simulink model "b747cl"  (Simulink 3.00)
settings: Solver=FixedStepDiscrete  StartTime=0.0  StopTime=Inf  RelTol=1e-3
libraries: simulink3 x2, airlib x1
settings Model: SaveTime=off  SaveOutput=off  ExtModeTrigMode=normal  ExtModeArmWhenConnect=on  LastModifiedBy=gcampa

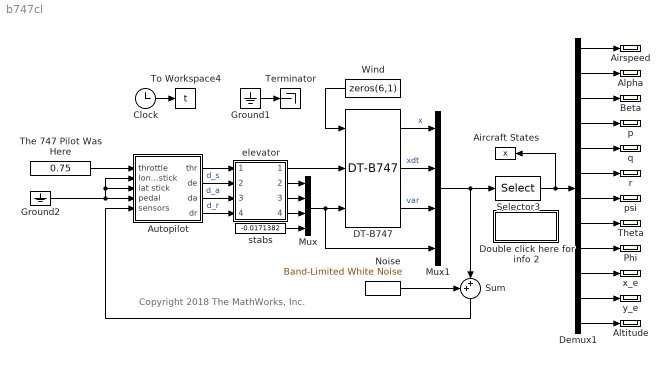
== system b747cl ==
  note: Copyright 2018 The MathWorks, Inc.
  Aircraft States : ToWorkspace  VariableName=x  SampleTime=0.05  SaveFormat=Matrix
      settings: Buffer=1000
  Airspeed : Scope
      settings: TimeRange=100  YMin=142.641  YMax=157.655  SaveToWorkspace=off  SaveName=ScopeData5
  Alpha : Scope
      settings: TimeRange=100  YMin=0.044176  YMax=0.0488262  SaveToWorkspace=off  SaveName=ScopeData4
  Altitude : Scope
      settings: TimeRange=100  YMin=57.9499  YMax=64.0499  SaveToWorkspace=off  SaveName=ScopeData15
  Autopilot : Subsystem
  Beta : Scope
      settings: TimeRange=100  YMin=0  YMax=250000  SaveToWorkspace=off  SaveName=ScopeData6
  Clock : Clock
      settings: DisplayTime=off  Decimation=10
  DT-B747 : airlib/DT-B747  GM1="[8.32   59.74   510.95   24675560  44876980   67383260   0   1315126  0   288772  0.05]"  CD_wind="[0.0164  0.2  0  0  0]"  CL_wind="[0.21  4.4  6.6  0.32  0.7]"  Cm_body="[0  -1   -20.5    -1.3    -2.7]"  CY_body="[0   -0.9    0     0     -0    0.12]"  Cl_body="[0    -0.16    -0.34   0.13    -0.013    0.008]"  Cn_body="[0    0.16   -0.026    -0.28     -0.0018   -0.1]"  x0="[150.148  0.0464959 0   0 0 0   0 0.0464959 0   0 0 61]"
  Demux1 : Demux  Outputs=12
  Double click here for info 2 : Subsystem
      mask Display: disp('Output\nSignals')
  Ground1 : Ground
  Ground2 : Ground
  Mux : Mux  Inputs=4
      settings: DisplayOption=none
  Mux1 : Mux  Inputs=[12 12 12 4]
      settings: DisplayOption=none
  Noise : simulink3/Sources/Band-Limited White Noise  Cov=[1e-7*ones(1,6) 1e-10*ones(1,3) zeros(1,31)]  Ts=0.05  seed=1:40
  Phi : Scope
      settings: TimeRange=100  YMin=-0.0002446  YMax=-0.0002438  SaveToWorkspace=off  SaveName=ScopeData12
  Selector3 : Selector  Elements=1:12  InputPortWidth=40
  Sum : Sum  Orientation=down  Inputs=++|  SaturateOnIntegerOverflow=on
  Terminator : Terminator
  The 747 Pilot Was Here : Constant  Value=0.75
  Theta : Scope
      settings: TimeRange=300  YMin=0.0463  YMax=0.0467  SaveToWorkspace=off  SaveName=ScopeData11
  To Workspace4 : ToWorkspace  VariableName=t  SampleTime=0.05  SaveFormat=Matrix
      settings: Buffer=1000
  Wind : Constant  Orientation=left  Value=zeros(6,1)
  elevator : Subsystem
      mask Display: disp('Cable &\nactuator\ndynamics')
  p : Scope
      settings: TimeRange=100  YMin=0  YMax=250000  SaveToWorkspace=off  SaveName=ScopeData7
  psi : Scope
      settings: TimeRange=100  YMin=0  YMax=250000  SaveToWorkspace=off  SaveName=ScopeData10
  q : Scope
      settings: TimeRange=100  YMin=0  YMax=250000  SaveToWorkspace=off  SaveName=ScopeData8
  r : Scope
      settings: TimeRange=100  YMin=0  YMax=250000  SaveToWorkspace=off  SaveName=ScopeData9
  stabs : Constant  Value=-0.0171382
  x_e : Scope
      settings: TimeRange=100  YMin=0  YMax=250000  SaveToWorkspace=off  SaveName=ScopeData13
  y_e : Scope
      settings: TimeRange=100  YMin=0  YMax=250000  SaveToWorkspace=off  SaveName=ScopeData14
  wires:
  elevator/3(deltaa) -> Mux/2
  elevator/4(deltar) -> Mux/3
  elevator/2(deltae) -> Mux/1
  Autopilot/2(de) -> elevator/2(D_elv)  "d_s"
  Autopilot/3(da) -> elevator/3(D_ail)  "d_a"
  Autopilot/4(dr) -> elevator/4(D_rud)  "d_r"
  Mux/1 -> Mux1/4, DT-B747/3
  elevator/1(throttle) -> DT-B747/2
  Mux1/1 -> Selector3/1, Sum/2
  Selector3/1 -> Demux1/1, Aircraft States/1
  Demux1/1 -> Airspeed/1
  Demux1/2 -> Alpha/1
  Demux1/3 -> Beta/1
  Demux1/4 -> p/1
  Demux1/5 -> q/1
  Demux1/6 -> r/1
  Demux1/7 -> psi/1
  Demux1/8 -> Theta/1
  Demux1/9 -> Phi/1
  Demux1/10 -> x_e/1
  Demux1/11 -> y_e/1
  Demux1/12 -> Altitude/1
  Autopilot/1(thr) -> elevator/1(D_thr)
  Clock/1 -> To Workspace4/1
  stabs/1 -> Mux/4
  Wind/1 -> DT-B747/1
  DT-B747/1 -> Mux1/1  "x"
  DT-B747/2 -> Mux1/2  "xdt"
  DT-B747/3 -> Mux1/3  "var"
  The 747 Pilot Was Here/1 -> Autopilot/1(throttle)
  Ground2/1 -> Autopilot/4(pedal), Autopilot/3(lat stick), Autopilot/2(long stick)
  Sum/1 -> Autopilot/5(sensors)
  Noise/1 -> Sum/1
  Ground1/1 -> Terminator/1

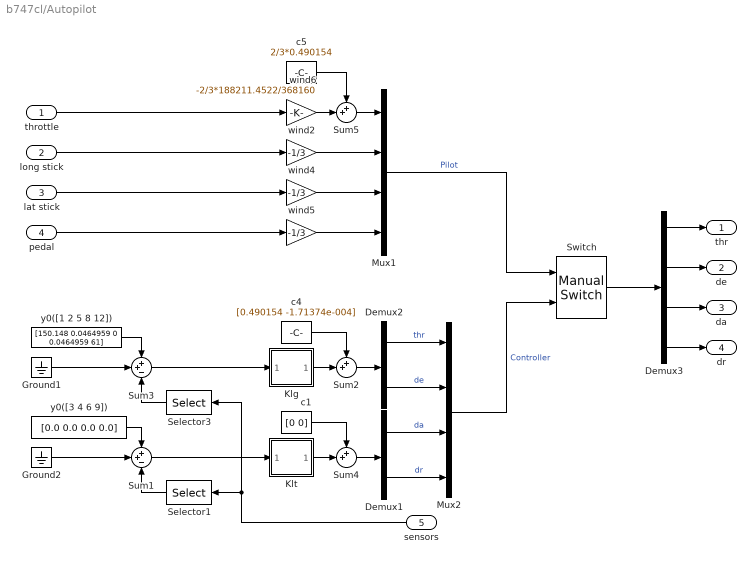
== system b747cl/Autopilot ==
  throttle : Inport  Port=1  PortWidth=-1  SampleTime=-1  DataType=auto
      settings: SignalType=auto
  long stick : Inport  Port=2  PortWidth=-1  SampleTime=-1  DataType=auto
      settings: SignalType=auto
  lat stick : Inport  Port=3  PortWidth=-1  SampleTime=-1  DataType=auto
      settings: SignalType=auto
  pedal : Inport  Port=4  PortWidth=-1  SampleTime=-1  DataType=auto
      settings: SignalType=auto
  sensors : Inport  Orientation=left  Port=5  PortWidth=-1  SampleTime=-1  DataType=auto
      settings: SignalType=auto
  Demux1 : Demux  Outputs=2
  Demux2 : Demux  Outputs=2
  Demux3 : Demux  Outputs=4
  Ground1 : Ground
  Ground2 : Ground
  "Klg " : Subsystem  mask(State Space){M=[0.1942   -0.8227    0.0057    0.6253    0.0090;  0.0283    7.9374   -5.0871  -16.2986   -0.0437]}
      mask prompts: M "Matrix"
      mask Display: disp('Matrix\nGain')
  "Klt " : Subsystem  mask(State Space){M=[0.2844   -0.1878   -0.2314   -0.1641; 1.1821   -0.4567   -1.8328   -0.4900]}
      mask prompts: M "Matrix"
      mask Display: disp('Matrix\nGain')
  Mux1 : Mux  Inputs=4
      settings: DisplayOption=none
  Mux2 : Mux  Inputs=4
      settings: DisplayOption=none
  Selector1 : Selector  Orientation=left  Elements=[3 4 6 9]  InputPortWidth=40
  Selector3 : Selector  Orientation=left  Elements=[1 2 5 8 12]  InputPortWidth=40
  Sum1 : Sum  Inputs=++-  SaturateOnIntegerOverflow=on
  Sum2 : Sum  Inputs=++|  SaturateOnIntegerOverflow=on
  Sum3 : Sum  Inputs=++-  SaturateOnIntegerOverflow=on
  Sum4 : Sum  Inputs=++|  SaturateOnIntegerOverflow=on
  Sum5 : Sum  Inputs=++|  SaturateOnIntegerOverflow=on
  Switch : simulink3/Nonlinear/Manual Switch  sw=0  action=0
  c1 : Constant  Value=[0 0]
  c4 : Constant  Value=[0.490154 -1.71374e-004]
  c5 : Constant  Value=2/3*0.490154
  wind2 : Gain  Gain=-1/3  SaturateOnIntegerOverflow=on
  wind4 : Gain  Gain=-1/3  SaturateOnIntegerOverflow=on
  wind5 : Gain  Gain=-1/3  SaturateOnIntegerOverflow=on
  wind6 : Gain  Gain=-2/3*188211.4522/368160  SaturateOnIntegerOverflow=on
  y0([1 2 5 8 12]) : Constant  Value="[150.148  0.0464959 0 0.0464959 61]"
  y0([3 4 6 9]) : Constant  Value=[0.0 0.0 0.0 0.0]
  thr : Outport  Port=1
  de : Outport  Port=2
  da : Outport  Port=3
  dr : Outport  Port=4
  wires:
  Selector1/1 -> Sum1/3
  Selector3/1 -> Sum3/3
  y0([3 4 6 9])/1 -> Sum1/1
  y0([1 2 5 8 12])/1 -> Sum3/1
  sensors/1 -> Selector1/1, Selector3/1
  Sum1/1 -> "Klt "/1(In1)
  Sum3/1 -> "Klg "/1(In1)
  Ground1/1 -> Sum3/2
  Ground2/1 -> Sum1/2
  Sum2/1 -> Demux2/1
  c4/1 -> Sum2/1
  long stick/1 -> wind2/1
  lat stick/1 -> wind4/1
  pedal/1 -> wind5/1
  Mux1/1 -> Switch/1  "Pilot"
  Demux1/1 -> Mux2/3  "da"
  Demux1/2 -> Mux2/4  "dr"
  Demux2/1 -> Mux2/1  "thr"
  Demux2/2 -> Mux2/2  "de"
  Switch/1 -> Demux3/1
  Demux3/1 -> thr/1
  Demux3/2 -> de/1
  Demux3/3 -> da/1
  Demux3/4 -> dr/1
  Mux2/1 -> Switch/2  "Controller"
  "Klg "/1(Out1) -> Sum2/2
  "Klt "/1(Out1) -> Sum4/2
  Sum4/1 -> Demux1/1
  c1/1 -> Sum4/1
  wind2/1 -> Mux1/2
  wind4/1 -> Mux1/3
  wind5/1 -> Mux1/4
  Sum5/1 -> Mux1/1
  throttle/1 -> wind6/1
  c5/1 -> Sum5/1
  wind6/1 -> Sum5/2

== system b747cl/Double click here for info 2 ==
  note: 01 v (m/s)
      | 02 alpha (rad)
      | 03 beta (rad)
      | 04 p (rad/s)
      | 05 q (rad/s)
      | 06 r  (rad/s)
      | 07 psi (rad)
      | 08 theta (rad)
      | 09 phi (rad)
      | 10 xe (m)
      | 11 ye (m)
      | 12 ze (m)
      | 13 v dot (m/s2)
      | 14 alpha dot (rad/s)
      | 15 beta dot (rad/s)
      | 16 p dot (rad/s2)
      | 17 q dot (rad/s2)
      | 18 r dot (rad/s2)
      | 19 fi dot (rad/s)
      | 20 theta dot (rad/s)
      | 21 psi dot (rad/s)
      | 22 xe dot (m/s)
      | 23 ye dot (m/s)
      | 24 ze dot (m/s)
      | 25 u dot (m/s2)
      | 26 v dot (m/s2)
      | 27 w dot (m/s2)
      | 28 pb/2v (rad)
      | 29 qc/v (rad)
      | 30 rb/v (rad)
      | 31 Ax (g)
      | 32 Ay (g)
      | 33 Az (g)
      | 34 ax (g)
      | 35 ay (g)
      | 36 az (g)
      | 37 delta elevators (rad)
      | 38 delta ailerons (rad)
      | 39 delta rudder (rad)
      | 40 delta stabs (rad)

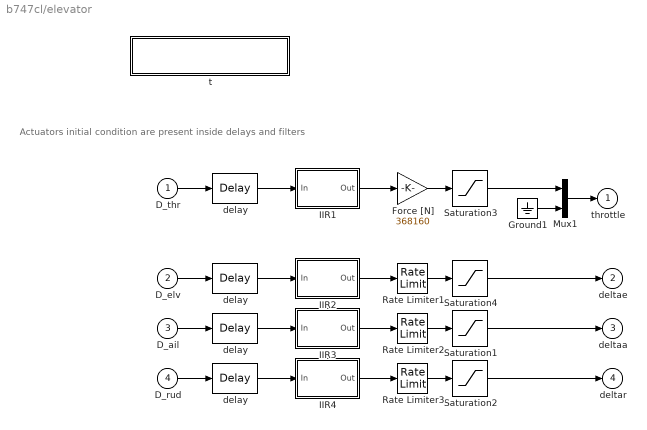
== system b747cl/elevator ==
  note: Actuators initial condition are present
      | inside delays and filters
  D_thr : Inport  Port=1  PortWidth=-1  SampleTime=-1  DataType=auto
      settings: SignalType=auto
  D_elv : Inport  Port=2  PortWidth=-1  SampleTime=-1  DataType=auto
      settings: SignalType=auto
  D_ail : Inport  Port=3  PortWidth=-1  SampleTime=-1  DataType=auto
      settings: SignalType=auto
  D_rud : Inport  Port=4  PortWidth=-1  SampleTime=-1  DataType=auto
      settings: SignalType=auto
  " delay" : TransportDelay  DelayTime=0.03  InitialInput=-1.71374e-004  BufferSize=1024
  " delay " : TransportDelay  DelayTime=0.03  InitialInput=0.490154  BufferSize=1024
  Force [N] : Gain  Gain=368160  SaturateOnIntegerOverflow=on
  Ground1 : Ground
  IIR1 : Subsystem  mask(Discrete Time First Order IIR){ni=1, a=4, x0=0.490154, T=0.05}
      mask prompts: ni "Number of Channels"; a "Cutoff Frequency (a)"; x0 "Initial Condition"; T "Sample Time"
      mask help:
      | Each channel has the transfer function
      |   (1-exp(-aT))/(1-exp(-aT)(z^-1)) which is a good
      |   (pz-matched) approximation of a/(s+a) if 10*a*T<pi
      mask init:
      | A=[];B=[];C=[];D=[];
      | for i=1:ni,
      | A=[A,zeros(size(A,1),1);zeros(1,size(A,2)),exp(-a*T)];
      | B=[B,zeros(size(B,1),1);zeros(1,size(B,2)),1-exp(-a*T)];
      | C=[C,zeros(size(C,1),1);zeros(1,size(C,2)),exp(-a*T)];
      | D=[D,zeros(size(D,1),1);zeros(1,size(D,2)),1-exp(-a*T)];
      | end
      mask Help:
      | <p>
      |   Each channel has the transfer function
      |   (1-exp(-aT))/(1-exp(-aT)(z^-1)) which is a good
      |   (pz-matched) approximation of a/(s+a) if 10*a*T<pi
      | </p>
      mask Display: dpoly(a,[1 a],'s')
  IIR2 : Subsystem  mask(Discrete Time First Order IIR){ni=1, a=15, x0=-1.71374e-004, T=0.05}
      mask prompts: ni "Number of Channels"; a "Cutoff Frequency (a)"; x0 "Initial Condition"; T "Sample Time"
      mask help:
      | Each channel has the transfer function
      |   (1-exp(-aT))/(1-exp(-aT)(z^-1)) which is a good
      |   (pz-matched) approximation of a/(s+a) if 10*a*T<pi
      mask init: same as b747cl/elevator/IIR1
      mask Help:
      | <p>
      |   Each channel has the transfer function
      |   (1-exp(-aT))/(1-exp(-aT)(z^-1)) which is a good
      |   (pz-matched) approximation of a/(s+a) if 10*a*T<pi
      | </p>
      mask Display: dpoly(a,[1 a],'s')
  IIR3 : Subsystem  mask(Discrete Time First Order IIR){ni=1, a=40, x0=0, T=0.05}
      mask prompts: ni "Number of Channels"; a "Cutoff Frequency (a)"; x0 "Initial Condition"; T "Sample Time"
      mask help:
      | Each channel has the transfer function
      |   (1-exp(-aT))/(1-exp(-aT)(z^-1)) which is a good
      |   (pz-matched) approximation of a/(s+a) if 10*a*T<pi
      mask init: same as b747cl/elevator/IIR1
      mask Help:
      | <p>
      |   Each channel has the transfer function
      |   (1-exp(-aT))/(1-exp(-aT)(z^-1)) which is a good
      |   (pz-matched) approximation of a/(s+a) if 10*a*T<pi
      | </p>
      mask Display: dpoly(a,[1 a],'s')
  IIR4 : Subsystem  mask(Discrete Time First Order IIR){ni=1, a=15, x0=0, T=0.05}
      mask prompts: ni "Number of Channels"; a "Cutoff Frequency (a)"; x0 "Initial Condition"; T "Sample Time"
      mask help:
      | Each channel has the transfer function
      |   (1-exp(-aT))/(1-exp(-aT)(z^-1)) which is a good
      |   (pz-matched) approximation of a/(s+a) if 10*a*T<pi
      mask init: same as b747cl/elevator/IIR1
      mask Help:
      | <p>
      |   Each channel has the transfer function
      |   (1-exp(-aT))/(1-exp(-aT)(z^-1)) which is a good
      |   (pz-matched) approximation of a/(s+a) if 10*a*T<pi
      | </p>
      mask Display: dpoly(a,[1 a],'s')
  Mux1 : Mux  Inputs=[1 5]
      settings: DisplayOption=none
  Rate Limiter1 : RateLimiter  RisingSlewLimit=100*pi/180  FallingSlewLimit=-100*pi/180
  Rate Limiter2 : RateLimiter  RisingSlewLimit=100*pi/180  FallingSlewLimit=-100*pi/180
  Rate Limiter3 : RateLimiter  RisingSlewLimit=100*pi/180  FallingSlewLimit=-100*pi/180
  Saturation1 : Saturate  UpperLimit=20*pi/180  LowerLimit=-20*pi/180
  Saturation2 : Saturate  UpperLimit=20*pi/180  LowerLimit=-20*pi/180
  Saturation3 : Saturate  UpperLimit=245440  LowerLimit=0
  Saturation4 : Saturate  UpperLimit=20*pi/180  LowerLimit=-20*pi/180
  delay : TransportDelay  DelayTime=0.03  InitialInput=0  BufferSize=1024
  "delay " : TransportDelay  DelayTime=0.03  InitialInput=0  BufferSize=1024
  t : Subsystem
      settings: OpenFcn=fdchelp actuatr
      mask Display: disp('Actuator & cable dynamics\nMarc Rauw, October 1997')
  throttle : Outport  Port=1
  deltae : Outport  Port=2
  deltaa : Outport  Port=3
  deltar : Outport  Port=4
  wires:
  D_ail/1 -> delay/1
  D_elv/1 -> " delay"/1
  D_rud/1 -> "delay "/1
  IIR2/1(Out) -> Rate Limiter1/1
  Saturation4/1 -> deltae/1
  IIR3/1(Out) -> Rate Limiter2/1
  Saturation1/1 -> deltaa/1
  IIR4/1(Out) -> Rate Limiter3/1
  Saturation2/1 -> deltar/1
  Rate Limiter1/1 -> Saturation4/1
  Rate Limiter2/1 -> Saturation1/1
  Rate Limiter3/1 -> Saturation2/1
  Mux1/1 -> throttle/1
  Saturation3/1 -> Mux1/1
  Ground1/1 -> Mux1/2
  D_thr/1 -> " delay "/1
  IIR1/1(Out) -> Force [N]/1
  Force [N]/1 -> Saturation3/1
  " delay "/1 -> IIR1/1(In)
  " delay"/1 -> IIR2/1(In)
  delay/1 -> IIR3/1(In)
  "delay "/1 -> IIR4/1(In)

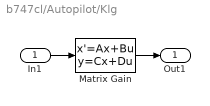
== system b747cl/Autopilot/Klg  ==
  In1 : Inport  Port=1  PortWidth=-1  SampleTime=-1  DataType=auto
      settings: SignalType=auto
  Matrix Gain : StateSpace  A=[]  B=[]  C=[]  D=M  X0=0
  Out1 : Outport  Port=1
  wires:
  In1/1 -> Matrix Gain/1
  Matrix Gain/1 -> Out1/1

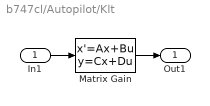
== system b747cl/Autopilot/Klt  ==
  In1 : Inport  Port=1  PortWidth=-1  SampleTime=-1  DataType=auto
      settings: SignalType=auto
  Matrix Gain : StateSpace  A=[]  B=[]  C=[]  D=M  X0=0
  Out1 : Outport  Port=1
  wires:
  In1/1 -> Matrix Gain/1
  Matrix Gain/1 -> Out1/1

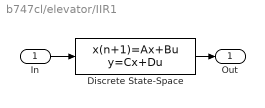
== system b747cl/elevator/IIR1 ==
  In : Inport  Port=1  PortWidth=-1  SampleTime=-1  DataType=auto
      settings: SignalType=auto
  Discrete State-Space : DiscreteStateSpace  A=A  B=B  C=C  D=D  X0=x0  SampleTime=T
  Out : Outport  Port=1
  wires:
  Discrete State-Space/1 -> Out/1
  In/1 -> Discrete State-Space/1

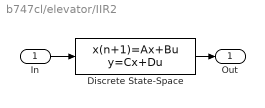
== system b747cl/elevator/IIR2 ==
  In : Inport  Port=1  PortWidth=-1  SampleTime=-1  DataType=auto
      settings: SignalType=auto
  Discrete State-Space : DiscreteStateSpace  A=A  B=B  C=C  D=D  X0=x0  SampleTime=T
  Out : Outport  Port=1
  wires:
  Discrete State-Space/1 -> Out/1
  In/1 -> Discrete State-Space/1

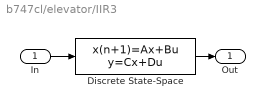
== system b747cl/elevator/IIR3 ==
  In : Inport  Port=1  PortWidth=-1  SampleTime=-1  DataType=auto
      settings: SignalType=auto
  Discrete State-Space : DiscreteStateSpace  A=A  B=B  C=C  D=D  X0=x0  SampleTime=T
  Out : Outport  Port=1
  wires:
  Discrete State-Space/1 -> Out/1
  In/1 -> Discrete State-Space/1

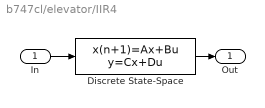
== system b747cl/elevator/IIR4 ==
  In : Inport  Port=1  PortWidth=-1  SampleTime=-1  DataType=auto
      settings: SignalType=auto
  Discrete State-Space : DiscreteStateSpace  A=A  B=B  C=C  D=D  X0=x0  SampleTime=T
  Out : Outport  Port=1
  wires:
  Discrete State-Space/1 -> Out/1
  In/1 -> Discrete State-Space/1

== system b747cl/elevator/t ==
